simulink model "sampleModel85"  (R2021b)
settings: Solver=VariableStepAuto  StartTime=0.0  StopTime=10.0  RelTol=1e-3
undefined symbols (not defined in the file or in its folder): DiscIntNeverNeededParam
libraries: simulink x15, slpidlib x1
settings Model: Creator=user  LastModifiedBy=user

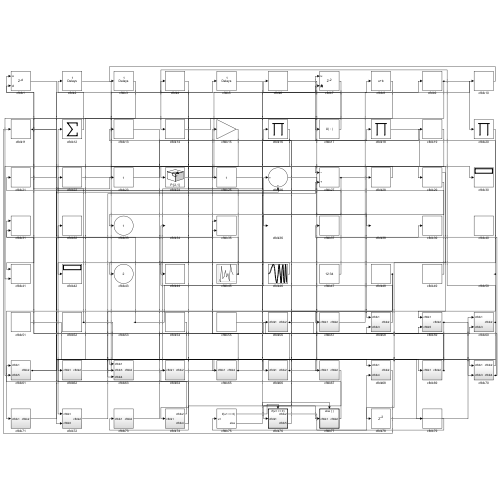
[thumbnail: Simulink's stored preview of the top-level diagram]
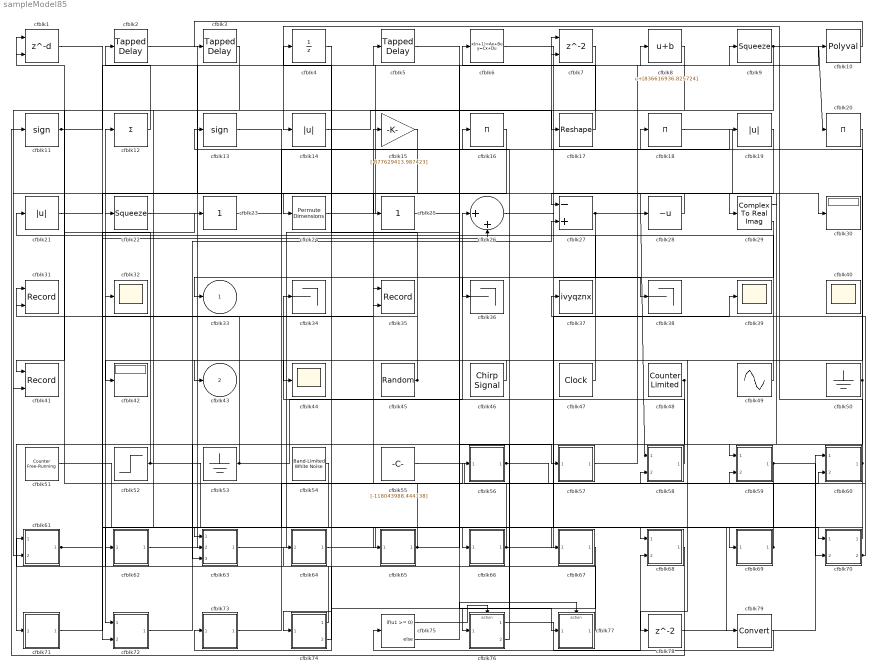
== system sampleModel85 ==
  cfblk1 : Delay  DelayLengthSource=Input port  SampleTime=1
      settings: InputPortMap=u0,p1
  cfblk10 : Polyval  Coefs=[ +2.081618890e-019, -1.441693666e-014, +4.719686976e-010, -8.536869453e-006, +1.621573104e-001, -8.087801117e+001 ]
  cfblk11 : Signum
  cfblk12 : Sum  Inputs=+
  cfblk13 : Signum
  cfblk14 : Abs
  cfblk15 : Gain  Gain=[-877629413.987423]
  cfblk16 : Product  Inputs=*
  cfblk17 : Reshape
  cfblk18 : Product  Inputs=*
  cfblk19 : Abs
  cfblk2 : simulink/Discrete/Tapped Delay  vinit=0.0  samptime=-1  NumDelays=1  DelayOrder=Oldest  includeCurrent=off
  cfblk20 : Product  Inputs=*
  cfblk21 : Abs
  cfblk22 : Squeeze
  cfblk23 : simulink/Math Operations/Slider Gain  gain=1  low=0  high=2
  cfblk24 : PermuteDimensions
  cfblk25 : simulink/Math Operations/Slider Gain  gain=1  low=0  high=2
  cfblk26 : Sum  Inputs=|++
  cfblk27 : Sum  Inputs=-+
  cfblk28 : UnaryMinus
  cfblk29 : ComplexToRealImag
  cfblk3 : simulink/Discrete/Tapped Delay  vinit=0.0  samptime=-1  NumDelays=1  DelayOrder=Oldest  includeCurrent=off
  cfblk30 : Display
  cfblk31 : Record  FileSettingsInternal="{\"entries\":[{\"content\":{\"excelSettings\":{\"content\":{},\"type\":\"Streamout.ExcelSettings\"}},\"type\":\"Streamout.FileSettingStorage\",\"uuid\":\"85da69d3-c91d-4e9a-b968-7592da699f8a\"}],\"packageUris\":[\"http://schema.mathworks.com/mf0/streamout_blocks/R2020a\"],\"version\":\"1.0\"}"  Layout=[1 1]  SignalsInternal="{\"entries\":[{\"content\":{\"signals\":[{\"content\":{\"blockPath\":[\"sampleModel85/cfblk31\"],\"channel\":[],\"dimensions\":[1],\"domain\":\"sampleModel85/cfblk31\",\"lineColor\":\"#a2142f\",\"plots\":[1],\"port\":1,\"sid\":[\"\"],\"signalID\":3141,\"signalName\":\"cfblk69\"},\"type\":\"RecordBlkView.Signal\",\"uuid\":\"782775ad-88f4-4e6d-9ed2-9390a92aee19\"},{\"content\":{\"blockPath\":[\"sampleModel85/cfblk31\"],\"channel\":[],\"dimensions\":[1],\"domain\":\"sampleModel85/cfblk31\",\"lineColor\":\"#139fff\",\"plots\":[1],\"port\":2,\"sid\":[\"\"],\"signalID\":3145,\"signalName\":\"cfblk45\"},\"type\":\"RecordBlkView.Signal\",\"uuid\":\"5b478cc4-92ff-481b-aa29-6d728f543560\"}]},\"type\":\"RecordBlkView.InputSignals\",\"uuid\":\"8621be74-1f9e-4678-95bd-487042e82b8f\"}],\"packageUris\":[\"http://schema.mathworks.com/mf0/streamout_blocks/R2020a\"],\"version\":\"1.0\"}"  VisualizationBindings="{\"xyplotplugin\":{\"info\":[{\"series\":[{\"bindingParametersList\":[{\"parameter\":\"X-Axis\",\"signalID\":3141,\"signalName\":\"cfblk69\"},{\"parameter\":\"Y-Axis\",\"signalID\":3145,\"signalName\":\"cfblk45\"}],\"seriesID\":42826}],\"subplotID\":1}]}}"  CompatibilityTag=XY
  cfblk{32,39..40,44} (4 alike) : Scope
      cfblk40 settings: Floating=on
  cfblk34 : Terminator
  cfblk35 : Record  FileSettingsInternal="{\"entries\":[{\"content\":{\"excelSettings\":{\"content\":{},\"type\":\"Streamout.ExcelSettings\"}},\"type\":\"Streamout.FileSettingStorage\",\"uuid\":\"0945f87c-6909-46fb-b5ad-a19f81f9b472\"}],\"packageUris\":[\"http://schema.mathworks.com/mf0/streamout_blocks/R2020a\"],\"version\":\"1.0\"}"  Layout=[1 1]  SignalsInternal="{\"entries\":[{\"content\":{\"signals\":[{\"content\":{\"blockPath\":[\"sampleModel85/cfblk35\"],\"channel\":[],\"dimensions\":[1],\"domain\":\"sampleModel85/cfblk35\",\"lineColor\":\"#a2142f\",\"plots\":[1],\"port\":1,\"sid\":[\"\"],\"signalID\":3149,\"signalName\":\"cfblk61\"},\"type\":\"RecordBlkView.Signal\",\"uuid\":\"17b30170-82dc-4401-b5a4-073c629dbdd3\"},{\"content\":{\"blockPath\":[\"sampleModel85/cfblk35\"],\"channel\":[],\"dimensions\":[1],\"domain\":\"sampleModel85/cfblk35\",\"lineColor\":\"#139fff\",\"plots\":[1],\"port\":2,\"sid\":[\"\"],\"signalID\":3153,\"signalName\":\"cfblk65\"},\"type\":\"RecordBlkView.Signal\",\"uuid\":\"3e5ecece-c173-45ad-bf85-157249e03370\"}]},\"type\":\"RecordBlkView.InputSignals\",\"uuid\":\"850d2042-2422-492f-8bc6-5e2a72413e86\"}],\"packageUris\":[\"http://schema.mathworks.com/mf0/streamout_blocks/R2020a\"],\"version\":\"1.0\"}"  VisualizationBindings="{\"xyplotplugin\":{\"info\":[{\"series\":[{\"bindingParametersList\":[{\"parameter\":\"X-Axis\",\"signalID\":3149,\"signalName\":\"cfblk61\"},{\"parameter\":\"Y-Axis\",\"signalID\":3153,\"signalName\":\"cfblk65\"}],\"seriesID\":14251}],\"subplotID\":1}]}}"  CompatibilityTag=XY
  cfblk36 : Terminator
  cfblk37 : ToWorkspace  VariableName=ivyqznx  SaveFormat=Timeseries  SampleTime=-1
  cfblk38 : Terminator
  cfblk4 : UnitDelay  HasFrameUpgradeWarning=on
  cfblk41 : Record  FileSettingsInternal="{\"entries\":[{\"content\":{\"excelSettings\":{\"content\":{},\"type\":\"Streamout.ExcelSettings\"}},\"type\":\"Streamout.FileSettingStorage\",\"uuid\":\"67b0c4ac-841f-43f6-9b18-6247b1b3d2c2\"}],\"packageUris\":[\"http://schema.mathworks.com/mf0/streamout_blocks/R2020a\"],\"version\":\"1.0\"}"  Layout=[1 1]  SignalsInternal="{\"entries\":[{\"content\":{\"signals\":[{\"content\":{\"blockPath\":[\"sampleModel85/cfblk41\"],\"channel\":[],\"dimensions\":[1],\"domain\":\"sampleModel85/cfblk41\",\"lineColor\":\"#a2142f\",\"plots\":[1],\"port\":1,\"sid\":[\"\"],\"signalID\":3157,\"signalName\":\"cfblk3\"},\"type\":\"RecordBlkView.Signal\",\"uuid\":\"b361bf5b-dc69-4bb2-8ea7-1953cfee71a2\"},{\"content\":{\"blockPath\":[\"sampleModel85/cfblk41\"],\"channel\":[],\"dimensions\":[1],\"domain\":\"sampleModel85/cfblk41\",\"lineColor\":\"#139fff\",\"plots\":[1],\"port\":2,\"sid\":[\"\"],\"signalID\":3161,\"signalName\":\"cfblk15\"},\"type\":\"RecordBlkView.Signal\",\"uuid\":\"19ef0a56-a73a-421d-85c1-b1235b4e4339\"}]},\"type\":\"RecordBlkView.InputSignals\",\"uuid\":\"a2b2bf91-3c74-4c9c-b8ad-59da7cb50384\"}],\"packageUris\":[\"http://schema.mathworks.com/mf0/streamout_blocks/R2020a\"],\"version\":\"1.0\"}"  VisualizationBindings="{\"xyplotplugin\":{\"info\":[{\"series\":[{\"bindingParametersList\":[{\"parameter\":\"X-Axis\",\"signalID\":3157,\"signalName\":\"cfblk3\"},{\"parameter\":\"Y-Axis\",\"signalID\":3161,\"signalName\":\"cfblk15\"}],\"seriesID\":60610}],\"subplotID\":1}]}}"  CompatibilityTag=XY
  cfblk42 : Display
  cfblk45 : UniformRandomNumber  Minimum=[-4554271486.154067]  Maximum=[8192892253.395101]  Seed=[87197993.000000]  SampleTime=0.1
  cfblk46 : simulink/Sources/Chirp Signal  f1=[642375875.172213]  T=[561319655.161188]  f2=[766435501.678711]
  cfblk47 : DigitalClock
  cfblk48 : simulink/Sources/Counter Limited  uplimit=[32.000000]  tsamp=-1
  cfblk49 : Sin  Amplitude=[964259925.849161]  Bias=[756577625.975215]  SampleTime=0
  cfblk5 : simulink/Discrete/Tapped Delay  vinit=0.0  samptime=-1  NumDelays=1  DelayOrder=Oldest  includeCurrent=off
  cfblk50 : Ground
  cfblk51 : simulink/Sources/Counter Free-Running  NumBits=[39.000000]  tsamp=-1
  cfblk52 : Step  Time=[35.000000]  Before=[897489262.276996]  After=[-135812818.810877]  SampleTime=0
  cfblk53 : Ground
  cfblk54 : simulink/Sources/Band-Limited White Noise  Cov=[9111983135.935801]  Ts=0.1  seed=[9831599024.000000]
  cfblk55 : Constant  Value=[-118043988.444138]  SampleTime=1
  cfblk56 : Subsystem
  cfblk57 : Subsystem
  cfblk58 : Subsystem
  cfblk59 : Subsystem
  cfblk6 : DiscreteStateSpace
  cfblk60 : Subsystem
  cfblk61 : Subsystem
  cfblk62 : Subsystem
  cfblk63 : Subsystem
  cfblk64 : Subsystem
  cfblk65 : Subsystem
  cfblk66 : Subsystem
  cfblk67 : Subsystem
  cfblk68 : Subsystem
  cfblk69 : Subsystem
  cfblk7 : Delay  ShowEnablePort=on  SampleTime=1
      settings: InputPortMap=u0,e6
  cfblk70 : Subsystem
  cfblk71 : Subsystem
  cfblk72 : Subsystem
  cfblk73 : Subsystem
  cfblk74 : Subsystem
  cfblk75 : If  IfExpression=u1 >= 0  SampleTime=1
  cfblk76 : Subsystem  TreatAsAtomicUnit=on
  cfblk77 : Subsystem  TreatAsAtomicUnit=on
  cfblk78 : Delay  SampleTime=1
  cfblk79 : DataTypeConversion
  cfblk8 : Bias  Bias=[836616936.825724]
  cfblk9 : Squeeze
  cfblk33 : Outport
  cfblk43 : Outport  Port=2
  wires:
  cfblk74/1(cfblk2) -> cfblk12/1
  cfblk52/1 -> cfblk70/1(cfblk1), cfblk1/1
  cfblk12/1 -> cfblk2/1
  cfblk49/1 -> cfblk21/1
  cfblk2/1 -> cfblk59/1(cfblk1)
  cfblk53/1 -> cfblk26/1, cfblk32/1
  cfblk16/1 -> cfblk24/1
  cfblk66/1(cfblk2) -> cfblk39/1, cfblk1/2
  cfblk67/1(cfblk2) -> cfblk73/1(cfblk1)
  cfblk48/1 -> cfblk71/1(cfblk1), cfblk63/2(cfblk3)
  cfblk4/1 -> cfblk74/1(cfblk1)
  cfblk55/1 -> cfblk59/2(cfblk5)
  cfblk60/1(cfblk2) -> cfblk14/1, cfblk63/3(cfblk4)
  cfblk6/1 -> cfblk68/1(cfblk1)
  cfblk54/1 -> cfblk72/1(cfblk1)
  cfblk47/1 -> cfblk22/1
  cfblk17/1 -> cfblk6/1
  cfblk71/1(cfblk2) -> cfblk26/2
  cfblk62/1(cfblk2) -> cfblk8/1
  cfblk9/1 -> cfblk20/1, cfblk44/1
  cfblk64/1(cfblk2) -> cfblk66/1(cfblk1)
  cfblk7/1 -> cfblk62/1(cfblk1)
  cfblk27/1 -> cfblk58/1(cfblk1), cfblk33/1
  cfblk50/1 -> cfblk7/1, cfblk76/1(cfblk1)
  cfblk11/1 -> cfblk65/1(cfblk1), cfblk5/1
  cfblk76/1(cfblk2) -> cfblk68/2(cfblk4)
  cfblk24/1 -> cfblk7/2
  cfblk13/1 -> cfblk69/1(cfblk1)
  cfblk70/1(cfblk2) -> cfblk63/1(cfblk1)
  cfblk19/1 -> cfblk28/1
  cfblk70/2(cfblk4) -> cfblk58/2(cfblk3), cfblk37/1
  cfblk65/1(cfblk2) -> cfblk18/1, cfblk35/2
  cfblk26/1 -> cfblk38/1
  cfblk29/1 -> cfblk42/1
  cfblk5/1 -> cfblk57/1(cfblk1)
  cfblk57/1(cfblk2) -> cfblk10/1
  cfblk22/1 -> cfblk29/1
  cfblk69/1(cfblk2) -> cfblk15/1, cfblk31/1
  cfblk73/1(cfblk2) -> cfblk56/1(cfblk1)
  cfblk68/1(cfblk2) -> cfblk11/1
  cfblk45/1 -> cfblk4/1, cfblk31/2
  cfblk56/1(cfblk2) -> cfblk16/1, cfblk60/2(cfblk3)
  cfblk76/2(cfblk5) -> cfblk13/1
  cfblk74/2(cfblk4) -> cfblk61/1(cfblk1)
  cfblk1/1 -> cfblk67/1(cfblk1)
  cfblk18/1 -> cfblk30/1
  cfblk63/1(cfblk2) -> cfblk9/1
  cfblk25/1 -> cfblk77/1(cfblk1)
  cfblk29/2 -> cfblk36/1
  cfblk28/1 -> cfblk27/1
  cfblk23/1 -> cfblk19/1
  cfblk21/1 -> cfblk25/1
  cfblk72/1(cfblk2) -> cfblk27/2
  cfblk10/1 -> cfblk3/1
  cfblk59/1(cfblk2) -> cfblk70/2(cfblk3), cfblk72/2(cfblk3)
  cfblk14/1 -> cfblk17/1
  cfblk3/1 -> cfblk41/1
  cfblk46/1 -> cfblk43/1
  cfblk58/1(cfblk2) -> cfblk34/1
  cfblk77/1(cfblk2) -> cfblk64/1(cfblk1)
  cfblk8/1 -> cfblk61/2(cfblk5)
  cfblk15/1 -> cfblk41/2
  cfblk61/1(cfblk2) -> cfblk35/1, cfblk23/1
  cfblk75/1 -> cfblk76/Action
  cfblk75/2 -> cfblk77/Action
  cfblk20/1 -> cfblk78/1
  cfblk78/1 -> cfblk60/1(cfblk1)
  cfblk51/1 -> cfblk79/1
  cfblk79/1 -> cfblk75/1

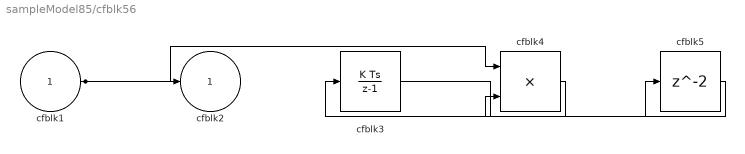
== system sampleModel85/cfblk56 ==
  cfblk1 : Inport
  cfblk3 : DiscreteIntegrator  ICPrevOutput=DiscIntNeverNeededParam  ICPrevScaledInput=DiscIntNeverNeededParam
  cfblk4 : Product
  cfblk5 : Delay  SampleTime=1
  cfblk2 : Outport
  wires:
  cfblk1/1 -> cfblk4/1, cfblk2/1
  cfblk4/1 -> cfblk3/1
  cfblk3/1 -> cfblk5/1
  cfblk5/1 -> cfblk4/2

== system sampleModel85/cfblk57 ==
  cfblk1 : Inport
  cfblk3 : Bias  Bias=[534578722.717567]
  cfblk2 : Outport
  wires:
  cfblk1/1 -> cfblk2/1, cfblk3/1

== system sampleModel85/cfblk58 ==
  cfblk1 : Inport
  cfblk3 : Inport  Port=2
  cfblk2 : Outport
  wires:
  cfblk3/1 -> cfblk2/1

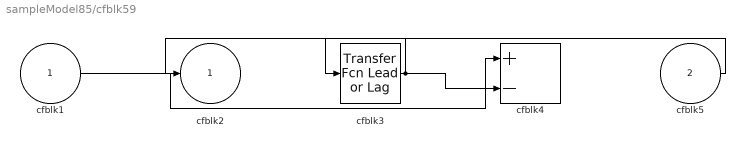
== system sampleModel85/cfblk59 ==
  cfblk1 : Inport
  cfblk5 : Inport  Port=2
  cfblk3 : simulink/Discrete/Transfer Fcn Lead or Lag  PoleZ=0.95  ZeroZ=0.75  ICPrevOutput=0.0  ICPrevInput=0.0  DoSatur=off
      settings: SourceProductBaseCode=SL
  cfblk4 : Sum  Inputs=+-
  cfblk2 : Outport
  wires:
  cfblk5/1 -> cfblk3/1
  cfblk1/1 -> cfblk4/1
  cfblk3/1 -> cfblk2/1, cfblk4/2

== system sampleModel85/cfblk60 ==
  cfblk1 : Inport
  cfblk3 : Inport  Port=2
  cfblk2 : Outport
  wires:
  cfblk1/1 -> cfblk2/1

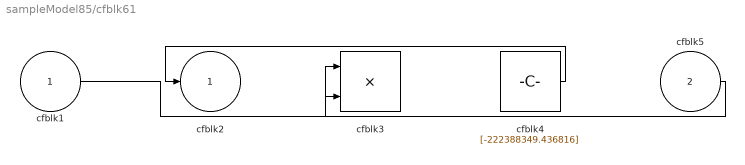
== system sampleModel85/cfblk61 ==
  cfblk1 : Inport
  cfblk5 : Inport  Port=2
  cfblk3 : Product  Inputs=**
  cfblk4 : Constant  Value=[-222388349.436816]  SampleTime=1
  cfblk2 : Outport
  wires:
  cfblk4/1 -> cfblk2/1
  cfblk5/1 -> cfblk3/1
  cfblk1/1 -> cfblk3/2

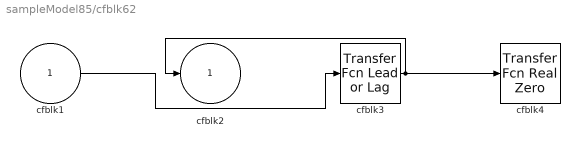
== system sampleModel85/cfblk62 ==
  cfblk1 : Inport
  cfblk3 : simulink/Discrete/Transfer Fcn Lead or Lag  PoleZ=0.95  ZeroZ=0.75  ICPrevOutput=0.0  ICPrevInput=0.0  DoSatur=off
      settings: SourceProductBaseCode=SL
  cfblk4 : simulink/Discrete/Transfer Fcn Real Zero  ZeroZ=0.75  ICPrevInput=0.0  DoSatur=off
      settings: SourceProductBaseCode=SL
  cfblk2 : Outport
  wires:
  cfblk3/1 -> cfblk2/1, cfblk4/1
  cfblk1/1 -> cfblk3/1

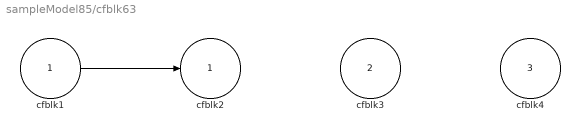
== system sampleModel85/cfblk63 ==
  cfblk1 : Inport
  cfblk3 : Inport  Port=2
  cfblk4 : Inport  Port=3
  cfblk2 : Outport
  wires:
  cfblk1/1 -> cfblk2/1

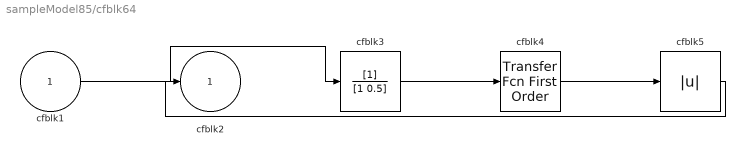
== system sampleModel85/cfblk64 ==
  cfblk1 : Inport
  cfblk3 : DiscreteFilter  SampleTime=1
  cfblk4 : simulink/Discrete/Transfer Fcn First Order  PoleZ=0.95  ICPrevOutput=0.0  DoSatur=off
  cfblk5 : Abs
  cfblk2 : Outport
  wires:
  cfblk4/1 -> cfblk5/1
  cfblk3/1 -> cfblk4/1
  cfblk1/1 -> cfblk3/1
  cfblk5/1 -> cfblk2/1

== system sampleModel85/cfblk65 ==
  cfblk1 : Inport
  cfblk3 : Abs
  cfblk2 : Outport
  wires:
  cfblk1/1 -> cfblk3/1
  cfblk3/1 -> cfblk2/1

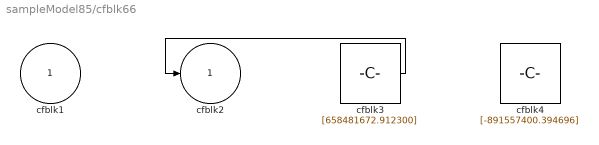
== system sampleModel85/cfblk66 ==
  cfblk1 : Inport
  cfblk3 : Constant  Value=[658481672.912300]  SampleTime=1
  cfblk4 : Constant  Value=[-891557400.394696]  SampleTime=1
  cfblk2 : Outport
  wires:
  cfblk3/1 -> cfblk2/1

== system sampleModel85/cfblk67 ==
  cfblk1 : Inport
  cfblk3 : DiscreteZeroPole  Poles=[0 0.5]  Gain=1
  cfblk2 : Outport
  wires:
  cfblk1/1 -> cfblk3/1
  cfblk3/1 -> cfblk2/1

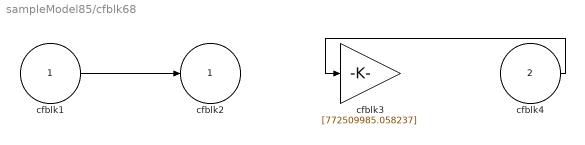
== system sampleModel85/cfblk68 ==
  cfblk1 : Inport
  cfblk4 : Inport  Port=2
  cfblk3 : Gain  Gain=[772509985.058237]
  cfblk2 : Outport
  wires:
  cfblk1/1 -> cfblk2/1
  cfblk4/1 -> cfblk3/1

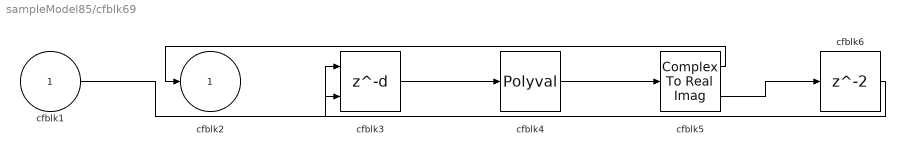
== system sampleModel85/cfblk69 ==
  cfblk1 : Inport
  cfblk3 : Delay  DelayLengthSource=Input port  SampleTime=1
      settings: InputPortMap=u0,p1
  cfblk4 : Polyval  Coefs=[ +2.081618890e-019, -1.441693666e-014, +4.719686976e-010, -8.536869453e-006, +1.621573104e-001, -8.087801117e+001 ]
  cfblk5 : ComplexToRealImag
  cfblk6 : Delay  SampleTime=1
  cfblk2 : Outport
  wires:
  cfblk5/1 -> cfblk2/1
  cfblk1/1 -> cfblk3/1
  cfblk4/1 -> cfblk5/1
  cfblk3/1 -> cfblk4/1
  cfblk5/2 -> cfblk6/1
  cfblk6/1 -> cfblk3/2

== system sampleModel85/cfblk70 ==
  cfblk1 : Inport
  cfblk3 : Inport  Port=2
  cfblk2 : Outport
  cfblk4 : Outport  Port=2
  wires:
  cfblk3/1 -> cfblk4/1
  cfblk1/1 -> cfblk2/1

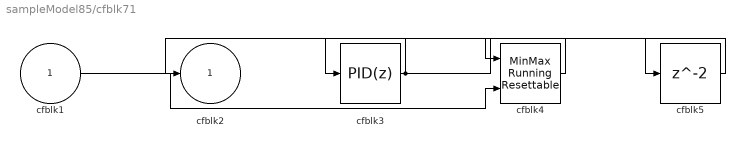
== system sampleModel85/cfblk71 ==
  cfblk1 : Inport
  cfblk3 : slpidlib/PID Controller  Controller=PID  Form=Parallel  TimeDomain=Discrete-time  UseExternalTs=off  SampleTime=1  IntegratorMethod=Forward Euler  FilterMethod=Forward Euler  ControllerParametersSource=internal  P=1  I=1  D=0  UseFilter=on  N=100  TunerSelectOption=Transfer Function Based (PID Tuner App)  InitialConditionSource=internal  InitialConditionForIntegrator=0  InitialConditionForFilter=0  DifferentiatorICPrevScaledInput=0  ExternalReset=none  TrackingMode=off  Kt=1  LimitOutput=off  SatLimitsSource=internal  UpperSaturationLimit=inf  LowerSaturationLimit=-inf  LinearizeAsGain=off  AntiWindupMode=none  Kb=1  POutMin=[]  POutMax=[]  IOutMin=[]  IOutMax=[]  DOutMin=[]  DOutMax=[]  NOutMin=[]  NOutMax=[]  SumOutMin=[]  SumOutMax=[]  SaturationOutMin=[]  SaturationOutMax=[]  PParamMin=[]  PParamMax=[]  IParamMin=[]  IParamMax=[]  DParamMin=[]  DParamMax=[]  NParamMin=[]  NParamMax=[]  KbParamMin=[]  KbParamMax=[]  KtParamMin=[]  KtParamMax=[]  KbOutMin=[]  KbOutMax=[]  KtOutMin=[]  KtOutMax=[]  IntegratorOutMin=[]  IntegratorOutMax=[]  FilterOutMin=[]  FilterOutMax=[]  SumI1OutMin=[]  SumI1OutMax=[]  SumI2OutMin=[]  SumI2OutMax=[]  SumI3OutMin=[]  SumI3OutMax=[]  SumI4OutMin=[]  SumI4OutMax=[]  SumDOutMin=[]  SumDOutMax=[]  DifferentiatorOutMin=[]  DifferentiatorOutMax=[]  FilterDiffOutCoefMin=[]  FilterDiffOutCoefMax=[]  ReciprocalOutMin=[]  ReciprocalOutMax=[]  SumDenOutMin=[]  SumDenOutMax=[]  SumNumOutMin=[]  SumNumOutMax=[]  DivideOutMin=[]  DivideOutMax=[]  UdiffTsProdOutMin=[]  UdiffTsProdOutMax=[]  NTsProdOutMin=[]  NTsProdOutMax=[]  UintegralTsProdOutMin=[]  UintegralTsProdOutMax=[]  UngainTsProdOutMin=[]  UngainTsProdOutMax=[]  IntegratorContinuousStateAttributes=''  IntegratorStateMustResolveToSignalObject=off  IntegratorRTWStateStorageClass=Auto  FilterContinuousStateAttributes=''  FilterStateMustResolveToSignalObject=off  FilterRTWStateStorageClass=Auto  ParallelPVariant=InternalParameters  IdealPVariant=Disabled  IVariant=InternalParameters  DVariant=InternalParameters  IntegratorVariant=Discrete  SatVariant=Disabled  AWVariant=Passthrough  PCopyVariant=Disabled  TRVariant=Disabled  FdbkBlocksVariant=Forward  IdealPFdbkVariant=Disabled  SatFdbkVariant=Disabled  DerivativeFilterVariant=ForwardEulerFilter  NVariant=InternalParameters  NCopyVariant=Disabled  FilterICVariant=InternalICsFilter  IntegratorICVariant=InternalICs  ExternalResetVariant=Disabled  TRSumVariant=Passthrough  SumFdbkVariant=Disabled  SumVariant=Sum_PID  TsampFilterVariant=InternalTs  TsampNgainVariant=Passthrough  TsampIntegralVariant=Passthrough  ExternalSaturationOutDataTypeStr=Inherit: Same as second input
  cfblk4 : simulink/Math Operations/MinMax Running Resettable  Function=min  vinit=0.0
  cfblk5 : Delay  SampleTime=1
  cfblk2 : Outport
  wires:
  cfblk4/1 -> cfblk3/1
  cfblk3/1 -> cfblk2/1, cfblk5/1
  cfblk1/1 -> cfblk4/2
  cfblk5/1 -> cfblk4/1

== system sampleModel85/cfblk72 ==
  cfblk1 : Inport
  cfblk3 : Inport  Port=2
  cfblk2 : Outport
  wires:
  cfblk1/1 -> cfblk2/1

== system sampleModel85/cfblk73 ==
  cfblk1 : Inport
  cfblk3 : MinMax  Function=max
  cfblk2 : Outport
  wires:
  cfblk1/1 -> cfblk3/1
  cfblk3/1 -> cfblk2/1

== system sampleModel85/cfblk74 ==
  cfblk1 : Inport
  cfblk3 : Constant  Value=[815722630.955212]  SampleTime=1
  cfblk2 : Outport
  cfblk4 : Outport  Port=2
  wires:
  cfblk1/1 -> cfblk4/1
  cfblk3/1 -> cfblk2/1

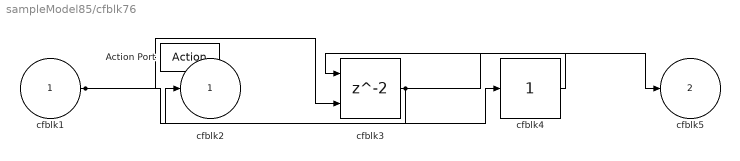
== system sampleModel85/cfblk76 ==
  cfblk1 : Inport
  Action Port : ActionPort  ActionPortLabel=if(u1 >= 0)
  cfblk3 : Delay  ShowEnablePort=on
      settings: InputPortMap=u0,e6
  cfblk4 : simulink/Math Operations/Slider Gain  gain=1  low=0  high=2
  cfblk2 : Outport
  cfblk5 : Outport  Port=2
  wires:
  cfblk3/1 -> cfblk2/1, cfblk5/1
  cfblk4/1 -> cfblk3/1
  cfblk1/1 -> cfblk3/2, cfblk4/1

== system sampleModel85/cfblk77 ==
  cfblk1 : Inport
  Action Port : ActionPort  ActionPortLabel=else
  cfblk3 : Sum  Inputs=|++
  cfblk2 : Outport
  wires:
  cfblk3/1 -> cfblk2/1
  cfblk1/1 -> cfblk3/1, cfblk3/2
